simulink model "Prelab1a_simulink_starter"  (R2019b)
settings: Solver=FixedStepDiscrete  StartTime=0.0  StopTime=50  FixedStep=5e-3  RelTol=1e-3  EnableMultiTasking=on
values from neighbouring files (symbols this model uses):
  A = (1-f)/T    (= 20)    [boone_submitting_extra_plotter.m]    (also in plotting_script_example.m)
  f = 0.9    [boone_submitting_extra_plotter.m]    (also in plotting_script_example.m)
  Kd = 1    [boone_submitting_extra_plotter.m]    (also in plotting_script_example.m)
  Kp = 10    [boone_submitting_extra_plotter.m]    (also in plotting_script_example.m = 100)
settings Model: Creator=katiebyl  LastModifiedBy=rboon
settings DataIOCC: ReturnWorkspaceOutputs=off
settings OptimizationCC: LifeSpan=inf
settings DebuggingCC: SFUnexpectedBacktrackingDiag=warning  SFNoUnconditionalDefaultTransitionDiag=warning  ArithmeticOperatorsInVariantConditions=warning
settings SFSimCC: SimUseLocalCustomCode=off  CustomCodeUndefinedFunction=UseInterfaceOnly
settings RTWCC: RTWUseLocalCustomCode=off  BuildConfiguration=Faster Runs
settings CodeAppCC: StateflowObjectComments=on
settings GRTTargetCC: TargetLangStandard=C89/C90 (ANSI)  GeneratePreprocessorConditionals=Disable all
settings ConfigComp: CovMetricSettings=dw  CovHtmlReporting=on  CovSaveCumulativeToWorkspaceVar=on  CovSaveSingleToWorkspaceVar=on  CovExternalEMLEnable=off

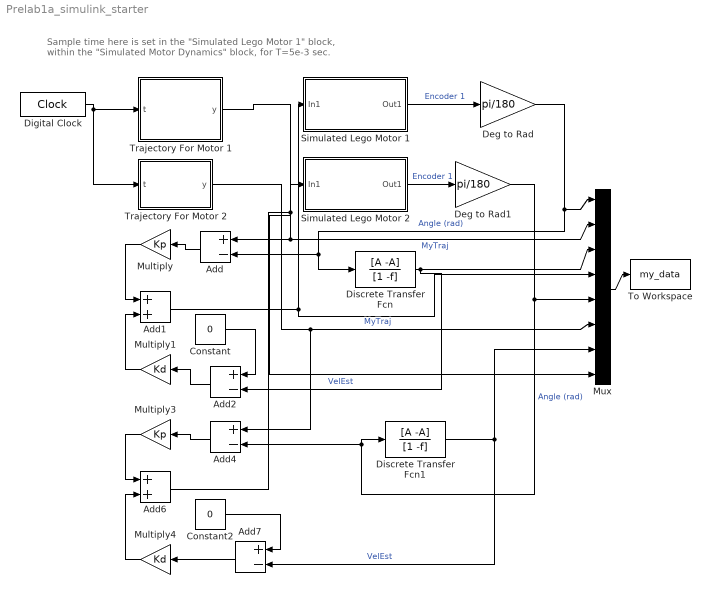
== system Prelab1a_simulink_starter ==
  note: Sample time here is set in the "Simulated Lego Motor 1" block,
      | within the "Simulated Motor Dynamics" block, for T=5e-3 sec.
  Add{,2,4,7} (4 alike) : Sum  Inputs=+-
  Add1 : Sum
  Add6 : Sum
  Constant : Constant  Value=0
  Constant2 : Constant  Value=0
  Deg to Rad : Gain  Gain=pi/180
  Deg to Rad1 : Gain  Gain=pi/180
  Digital Clock : DigitalClock  SampleTime=5e-3
  Discrete Transfer Fcn : DiscreteTransferFcn  Numerator=[A -A]  Denominator=[1 -f]  SampleTime=0.005
  Discrete Transfer Fcn1 : DiscreteTransferFcn  Numerator=[A -A]  Denominator=[1 -f]  SampleTime=0.005
  Multiply : Gain  Gain=Kp
  Multiply1 : Gain  Gain=Kd
  Multiply3 : Gain  Gain=Kp
  Multiply4 : Gain  Gain=Kd
  Mux : Mux  Inputs=8
  Simulated Lego Motor 1 : Subsystem
  Simulated Lego Motor 2 : Subsystem
  To Workspace : ToWorkspace  VariableName=my_data  SaveFormat=Structure With Time  SampleTime=-1
  Trajectory For Motor 1 : MATLAB Function  TreatAsAtomicUnit=on
  Trajectory For Motor 2 : MATLAB Function  TreatAsAtomicUnit=on
  wires:
  Simulated Lego Motor 1/1(Out1) -> Deg to Rad/1  "Encoder 1"
  Deg to Rad/1 -> Discrete Transfer Fcn/1, Add/2, Mux/1  "Angle (rad)"
  Mux/1 -> To Workspace/1
  Digital Clock/1 -> Trajectory For Motor 2/1(t), Trajectory For Motor 1/1(t)
  Trajectory For Motor 1/1(y) -> Add/1, Mux/2  "MyTraj"
  Trajectory For Motor 2/1(y) -> Add4/1, Mux/6  "MyTraj"
  Simulated Lego Motor 2/1(Out1) -> Deg to Rad1/1  "Encoder 1"
  Discrete Transfer Fcn/1 -> Mux/3, Add2/2  "VelEst"
  Add/1 -> Multiply/1
  Multiply1/1 -> Add1/2
  Multiply/1 -> Add1/1
  Add1/1 -> Simulated Lego Motor 1/1(In1), Mux/4
  Add2/1 -> Multiply1/1
  Constant/1 -> Add2/1
  Add7/1 -> Multiply4/1
  Constant2/1 -> Add7/1
  Multiply4/1 -> Add6/2
  Deg to Rad1/1 -> Mux/5, Discrete Transfer Fcn1/1, Add4/2  "Angle (rad)"
  Add4/1 -> Multiply3/1
  Multiply3/1 -> Add6/1
  Discrete Transfer Fcn1/1 -> Add7/2, Mux/7  "VelEst"
  Add6/1 -> Mux/8, Simulated Lego Motor 2/1(In1)

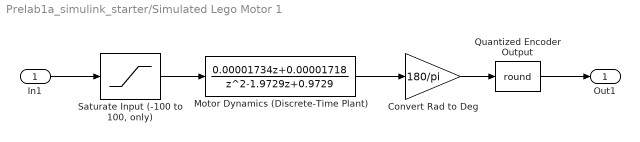
== system Prelab1a_simulink_starter/Simulated Lego Motor 1 ==
  In1 : Inport
  Convert Rad to Deg : Gain  Gain=180/pi
  Motor Dynamics (Discrete-Time Plant) : DiscreteTransferFcn  Numerator="[0.00001734  0.00001718]"  Denominator="[1   -1.9729    0.9729]"
  Quantized Encoder Output : Rounding  Operator=round
  "Saturate Input (-100 to 100, only)" : Saturate  UpperLimit=100  LowerLimit=-100
  Out1 : Outport
  wires:
  In1/1 -> "Saturate Input (-100 to 100, only)"/1
  "Saturate Input (-100 to 100, only)"/1 -> Motor Dynamics (Discrete-Time Plant)/1
  Convert Rad to Deg/1 -> Quantized Encoder Output/1
  Motor Dynamics (Discrete-Time Plant)/1 -> Convert Rad to Deg/1
  Quantized Encoder Output/1 -> Out1/1

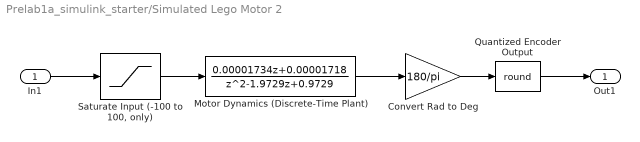
== system Prelab1a_simulink_starter/Simulated Lego Motor 2 ==
  In1 : Inport
  Convert Rad to Deg : Gain  Gain=180/pi
  Motor Dynamics (Discrete-Time Plant) : DiscreteTransferFcn  Numerator="[0.00001734  0.00001718]"  Denominator="[1   -1.9729    0.9729]"
  Quantized Encoder Output : Rounding  Operator=round
  "Saturate Input (-100 to 100, only)" : Saturate  UpperLimit=100  LowerLimit=-100
  Out1 : Outport
  wires:
  In1/1 -> "Saturate Input (-100 to 100, only)"/1
  "Saturate Input (-100 to 100, only)"/1 -> Motor Dynamics (Discrete-Time Plant)/1
  Convert Rad to Deg/1 -> Quantized Encoder Output/1
  Motor Dynamics (Discrete-Time Plant)/1 -> Convert Rad to Deg/1
  Quantized Encoder Output/1 -> Out1/1

== matlab function Prelab1a_simulink_starter/Trajectory For Motor 1 ==
  data: t input; y output

function y = MyTrajectory(t)
L1 = 14.5;
L2 = 10.5;
timetot = 10;
%% Define y(t) as a desired TRAJECTORY as a function of TIME
if 0
    h = 10 + 2.5*sqrt(3);
    ti = [0 10 12 22 24 34 36 46 200];
    xi = [7.5 7.5 12.5 12.5 10 10 7.5 7.5 7.5];
    yi = [10 10 10 10 h h 10 10 10];
    set = 0;
    y = 0;
    for i=1:8
        if ti(i) <= t && ti(i+1) > t
            set = 1;
            partdist = (t - ti(i))/(ti(i+1) - ti(i));
            xloc = (partdist * (xi(i+1) - xi(i))) + xi(i);
            yloc = (partdist * (yi(i+1) - yi(i))) + yi(i);
            y = TranslateToThetaOne(xloc, yloc, L1, L2);
        end
    end
    if set == 0
        y = 0;
    end
elseif 1
    %%Lab1b Prelab trajectory
    ytraj = [-2,   -2,   -2,   -2,   -2,   -2,   0,    1,    2,    3,    4,    5,    6,    7 ,   8,    9,    10,   11,   12,   13,   14,   15,   15,   15,   15,   15,   15,   15,  15,  15,  15,  15,  15,   14,   13,   12,   11,   10,   9,    8,    7,    6,    6,    6, 6, 6, 6,  6,  6,     7,     8,     9,     10,    11,    12,    12, 12, 12, 11.5, 11.25, 11, 11, 11, 11, 11, 11];
    xtraj = [15.5, 15.5, 15.5, 15.5, 15.5, 15.5, 15.5, 15.5, 15.5, 15.5, 15.5, 15.5, 15.5, 15.5, 15.5, 15.5, 15.5, 15.5, 15.5, 15.5, 15.5, 15.5, 14.5, 13.5, 12.5, 11.5, 10.5, 9.5, 8.5, 7.5, 6.5, 5.5, 4.75, 4.75, 4.75, 4.75, 4.75, 4.75, 4.75, 4.75, 4.75, 4.75, 5.75, 7, 8, 9, 10, 11, 12.25, 12.25, 12.25, 12.25, 12.25, 12.25, 12.25, 11, 10, 9,  8,    7,     6,  6,  6,  6,  6,  6];    timepoint = 0:timetot/70:timetot;
    for i=1:65
        if t >= timepoint(i) & t < timepoint(i+1)
            timediff = (t - timepoint(i))/(timepoint(i+1) - timepoint(i));
            xval = ((xtraj(i+1) - xtraj(i)) * timediff) + xtraj(i);
            yval = ((ytraj(i+1) - ytraj(i)) * timediff) + ytraj(i);
            break
        end
        xval = 15.5;
        yval = 0;
    end
    y = TranslateToThetaOne(xval, yval, L1, L2);
elseif 0
    %% Example 1: a step, which starts at t=1 second
    t_start = 1; % have the step occur at t = t_start
    StepMag = 0.3; % For a step in RAW INPUT to motor (open loop)
    % StepMag = 0.3; % for a step in RADIANS, as a TRAJECTORY (closed loop)
    % Here, this the VALUE TO THE MOTOR (analogous to open-loop voltage)
    if t>=t_start
        y = StepMag;
    else
        y = 0;
    end
    
    
elseif 0
    %% Example 2: a trajectory, in RADIANS, for the motor to follow
    t_start = 1;
    A = 0.3; % In RADIANS
    w = 2*2*pi;
    if t>=t_start
        t_use = t - t_start;
        y = A * sin(w*t_use);
    else
        y = 0;
    end
    
elseif 0
    %% Example 3: using interp1() and some waypoints
    ti = [0 1 2 3 100];
    yi = [0 0 20 -30 -30]*(pi/180);
    y = interp1(ti,yi,t);  % LINEAR INTERPOLATION, as a REFERENCE
else
    %% Example 4: using half-cosine function, for smooth transitions
    ypts = [0 0 30 -20 0 0]*pi/180;
    tpts = [0 1 2 3 4 10];
    if t < tpts(2)
        y1 = ypts(1); y2 = ypts(2);
        t1 = tpts(1); t2 = tpts(2);
    elseif t < tpts(3)
        y1 = ypts(2); y2 = ypts(3);
        t1 = tpts(2); t2 = tpts(3);
    elseif t < tpts(4)
        y1 = ypts(3); y2 = ypts(4);
        t1 = tpts(3); t2 = tpts(4);
    elseif t < tpts(5)
        y1 = ypts(4); y2 = ypts(5); % Hold at SAME VALUE
        t1 = tpts(4); t2 = tpts(5);
    else
        y1 = ypts(5); y2 = ypts(6);
        t1 = tpts(5); t2 = tpts(6);
    end
    tPhase = (t-t1) / (t2-t1);  % goes from 0 to 1
    cosVal = cos(pi * tPhase);  % cos(pi*tPhase) will go from 1 to -1...
    y = y1 + (y2 - y1) * (.5 * (1-cosVal)); % cosine shape, going
    % from 0 to 1, as tPhase goes from 0 to pi.
end
end



function theta_two = TranslateToThetaTwo(x, y, L1, L2)
    top =  ((x^2) + (y^2)) - (L1^2) -  (L2^2);
    bottom = 2 * L1 * L2;
    c = top/bottom;
%     s2 = sqrt(1 - (c^2));
%     theta_two =  pi - acos(top/bottom);
    theta_two = acos(c);
end

function theta_one = TranslateToThetaOne(x, y, L1, L2)
    theta_two = TranslateToThetaTwo(x, y, L1, L2);
    left = atan(y/x);
    right = atan((L2 * sin(theta_two))/(L1 + (L2 * cos(theta_two))));
    theta_one = left - right;
end

== matlab function Prelab1a_simulink_starter/Trajectory For Motor 2 ==
  data: t input; y output

function y = MyTrajectory(t)
L1 = 14.5;
L2 = 10.5;
timetot = 10;
%% Define y(t) as a desired TRAJECTORY as a function of TIME
if 0
    h = 10 + 2.5*sqrt(3);
    ti = [0 10 12 22 24 34 36 46 200];
    xi = [7.5 7.5 12.5 12.5 10 10 7.5 7.5 7.5];
    yi = [10 10 10 10 h h 10 10 10];
    set = 0;
    y = 0;
    for i=1:8
        if ti(i) <= t && ti(i+1) > t
            set = 1;
            partdist = (t - ti(i))/(ti(i+1) - ti(i));
            xloc = (partdist * (xi(i+1) - xi(i))) + xi(i);
            yloc = (partdist * (yi(i+1) - yi(i))) + yi(i);
            y = TranslateToThetaTwo(xloc, yloc, L1, L2);
        end
    end
    if set == 0
        y = 0;
    end    
    
elseif 0
    %% Example 1: a step, which starts at t=1 second
    t_start = 1; % have the step occur at t = t_start
    StepMag = 100; % For a step in RAW INPUT to motor (open loop)
    % StepMag = 0.3; % for a step in RADIANS, as a TRAJECTORY (closed loop)
    % Here, this the VALUE TO THE MOTOR (analogous to open-loop voltage)
    if t>=t_start
        y = StepMag;
    else
        y = 0;
    end
elseif 1
    %%Lab1b Prelab trajectory
    ytraj = [-2,   -2,   -2,   -2,   -2,   -2,   0,    1,    2,    3,    4,    5,    6,    7 ,   8,    9,    10,   11,   12,   13,   14,   15,   15,   15,   15,   15,   15,   15,  15,  15,  15,  15,  15,   14,   13,   12,   11,   10,   9,    8,    7,    6,    6,    6, 6, 6, 6,  6,  6,     7,     8,     9,     10,    11,    12,    12, 12, 12, 11.5, 11.25, 11, 11, 11, 11, 11, 11];
    xtraj = [15.5, 15.5, 15.5, 15.5, 15.5, 15.5, 15.5, 15.5, 15.5, 15.5, 15.5, 15.5, 15.5, 15.5, 15.5, 15.5, 15.5, 15.5, 15.5, 15.5, 15.5, 15.5, 14.5, 13.5, 12.5, 11.5, 10.5, 9.5, 8.5, 7.5, 6.5, 5.5, 4.75, 4.75, 4.75, 4.75, 4.75, 4.75, 4.75, 4.75, 4.75, 4.75, 5.75, 7, 8, 9, 10, 11, 12.25, 12.25, 12.25, 12.25, 12.25, 12.25, 12.25, 11, 10, 9,  8,    7,     6,  6,  6,  6,  6,  6];    timepoint = 0:timetot/70:timetot;
    for i=1:65
        if t >= timepoint(i) & t < timepoint(i+1)
            timediff = (t - timepoint(i))/(timepoint(i+1) - timepoint(i));
            xval = ((xtraj(i+1) - xtraj(i)) * timediff) + xtraj(i);
            yval = ((ytraj(i+1) - ytraj(i)) * timediff) + ytraj(i);
            break
        end
        xval = 15.5;
        yval = 0;
    end
    y = TranslateToThetaTwo(xval, yval, L1, L2);
    
elseif 0
    %% Example 2: a trajectory, in RADIANS, for the motor to follow
    t_start = 1;
    A = 0.3; % In RADIANS
    w = 2*2*pi;
    if t>=t_start
        t_use = t - t_start;
        y = A * sin(w*t_use);
    else
        y = 0;
    end
    
elseif 0
    %% Example 3: using interp1() and some waypoints
    ti = [0 1 2 3 100];
    yi = [0 0 20 -30 -30]*(pi/180);
    y = interp1(ti,yi,t);  % LINEAR INTERPOLATION, as a REFERENCE
else
    %% Example 4: using half-cosine function, for smooth transitions
    ypts = [0 0 30 -20 0 0]*pi/180;
    tpts = [0 1 2 3 4 10];
    if t < tpts(2)
        y1 = ypts(1); y2 = ypts(2);
        t1 = tpts(1); t2 = tpts(2);
    elseif t < tpts(3)
        y1 = ypts(2); y2 = ypts(3);
        t1 = tpts(2); t2 = tpts(3);
    elseif t < tpts(4)
        y1 = ypts(3); y2 = ypts(4);
        t1 = tpts(3); t2 = tpts(4);
    elseif t < tpts(5)
        y1 = ypts(4); y2 = ypts(5); % Hold at SAME VALUE
        t1 = tpts(4); t2 = tpts(5);
    else
        y1 = ypts(5); y2 = ypts(6);
        t1 = tpts(5); t2 = tpts(6);
    end
    tPhase = (t-t1) / (t2-t1);  % goes from 0 to 1
    cosVal = cos(pi * tPhase);  % cos(pi*tPhase) will go from 1 to -1...
    y = y1 + (y2 - y1) * (.5 * (1-cosVal)); % cosine shape, going
    % from 0 to 1, as tPhase goes from 0 to pi.
end
end




function theta_two = TranslateToThetaTwo(x, y, L1, L2)
    x
    y
    top =  ((x^2) + (y^2)) - (L1^2) -  (L2^2)
    bottom = 2 * L1 * L2
    c = top/bottom;
%     s2 = sqrt(1 - (c^2));
%     theta_two =  pi - acos(top/bottom);
    theta_two = acos(c);
end

function theta_one = TranslateToThetaOne(x, y, L1, L2)
    theta_two = TranslateToThetaTwo(x, y, L1, L2);
    left = atan(y/x);
    right = atan((L2 * sin(theta_two))/(L1 + (L2 * cos(theta_two))));
    theta_one = left - right;
end
